simulink model "vd_controller"  (R2019b)
settings: configuration reference "E9_ECU_Configuration" (kept outside this file)
undefined symbols (not defined in the file or in its folder): BrakeMap_default_breakpoints, BrakeMap_default_data, disable_9D_front, disable_slipanglesensor, mask_select_input_pGL, Sq_PosBadGradient, Sq_PosIsFrozen, Sq_PosOutOfBounds
libraries: SignalProcessingSensorFusionLib x38, simulink x30, hdlsllib x3
(part 1 of 2)
settings Model: DataDictionary=dd_MainControl.sldd  EnableAccessToBaseWorkspace=off  ExplicitPartitioning=on  Creator=chwit  LastModifiedBy=laura
settings Model: ModifiedComment=|
  | schwa -- Fri Mar 02 10:09:33 2018 -- Version 1.53
  | Switched names of ControlAllocation, minimal Version active
settings Model: ModifiedHistory=|
  | schwa -- Fri Mar 02 10:09:33 2018 -- Version 1.53
  | Switched names of ControlAllocation, minimal Version active
  | 
  | schwa -- Fri Mar 02 10:09:33 2018 -- Version 1.53
  | Switched names of ControlAllocation, minimal Version active
  | 
  | schwa -- Fri Mar 02 01:32:20 2018 -- Version 1.52
  | cosmetic changes, adjusted ports
  | 
  | schwa -- Fri Mar 02 01:28:29 2018 -- Version 1.51
  | 
  | schwa -- Fri Mar 02 01:26:02 2018 -- Version 1.50
  | integrated new FF
  | 
  | 
  | chwit -- Fri Feb 23 19:55:57 2018 -- Version 1.49
  | 
  | chwit -- Fri Feb 23 07:06:27 2018 -- Version 1.48
  | Buildable but yet not flashable version of initial version of ControlSystem for E9 after function freeze v1
  | 
  | 
  | 
  | chwit -- Sun Feb 18 18:12:23 2018 -- Version 1.20
  | 
  | chwit -- Sun Feb 18 18:12:23 2018 -- Version 1.20
  | 
  | chwit -- Sun Feb 18 18:02:59 2018 -- Version 1.19
  | 
  | chwit -- Sun Feb 18 17:57:29 2018 -- Version 1.18
  | Saving
  | 
  | 
  | chwit -- Sun Feb 18 17:09:51 2018 -- Version 1.17
  | Saving
  | 
  | chwit -- Sun Feb 18 17:09:04 2018 -- Version 1.16
  | Just for saving purposes
  | 
  | chwit -- Sun Feb 18 14:38:44 2018 -- Version 1.15
  | YawMoment -> YawAcc corrected
  | 
  | 
  | chwit -- Sun Feb 18 12:57:57 2018 -- Version 1.14
  | Function freeze and new structure
  | 
  | 
  | chwit -- Sun Feb 18 12:51:11 2018 -- Version 1.13
  | Changes made due to function freeze and new structure
  | 
  | 
  | chwit -- Sun Feb 18 11:51:16 2018 -- Version 1.11
  | Implemented Manual Mode
  | 
  | chwit -- Sun Feb 18 11:51:16 2018 -- Version 1.11
  | Implemented Manual Mode
  | 
  | Marko -- Sat Feb 17 23:21:38 2018 -- Version 1.10
  | Changed Subsystem ConvertToInverterSingals: Deleted Everything except kt-Kennlinie, added limit on TorqueRequest
  | 
  | added OverUndersteerCorrection between FF and CA, connected CA with temporary (dummy) signals until right signals are provided
  | schwa -- Wed Feb 14 10:07:50 2018 -- Version 1.9
  | 
  | rearranged signals
  | schwa -- Wed Feb 14 09:51:50 2018 -- Version 1.8
  | 
  | chwit -- Sat Jan 20 18:54:27 2018 -- Version 1.7
  | 
  | chwit -- Sat Jan 20 17:46:44 2018 -- Version 1.6
  | 
  | chwit -- Sat Jan 20 17:42:35 2018 -- Version 1.5
  | Initial version
settings ConfigSetRef: SourceName=E9_ECU_Configuration

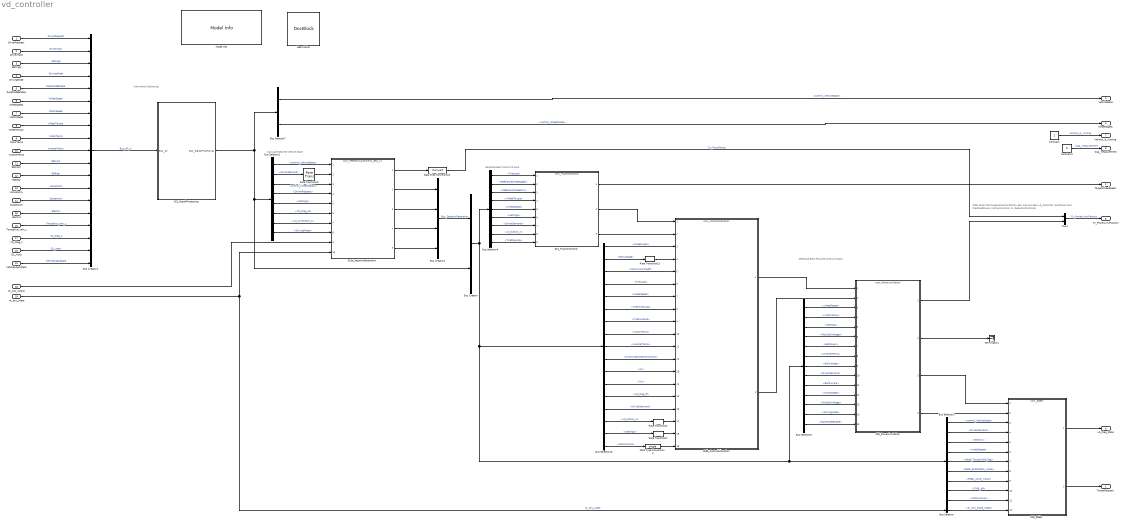
== system vd_controller ==
  note: ToDo: Einen Fahrzeugzustand einführen, den man aus dem
      |  vd_controller rausführen kann: PredictedPower, KalmanZustand, Fx, ReductionFaktoren
  note: Information Gathering
  note: Calculate Desired Vehicle State
  note: Generate Best Control Output
  note: Generate Best Possible Control Output
  DriverRequest : Inport  OutDataTypeStr=Bus: control_DriverRequest  SampleTime=0.01
  DriverInput : Inport  Port=2  OutDataTypeStr=Bus: control_DriverInput  SampleTime=0.1
  Settings : Inport  Port=3  OutDataTypeStr=Bus: control_Settings  SampleTime=0.1
  DrivingMode : Inport  Port=4  OutDataTypeStr=single  PortDimensions=1  SampleTime=0.1
  RaceModeEnable : Inport  Port=5  OutDataTypeStr=boolean  SampleTime=0.1
  WheelSpeed : Inport  Port=6  OutDataTypeStr=single  PortDimensions=4  SampleTime=0.001
  MotorSpeed : Inport  Port=7  OutDataTypeStr=single  PortDimensions=4  SampleTime=0.001
  WheelTorque : Inport  Port=8  OutDataTypeStr=single  PortDimensions=4  SampleTime=0.001
  MotorTemp : Inport  Port=9  OutDataTypeStr=single  PortDimensions=4  SampleTime=0.5
  InverterTemp : Inport  Port=10  OutDataTypeStr=single  PortDimensions=4  SampleTime=0.5
  9DFront : Inport  Port=11  OutDataTypeStr=Bus: control_9D  SampleTime=0.002
  9DRear : Inport  Port=12  OutDataTypeStr=Bus: control_9D  SampleTime=0.002
  v2oVelocity : Inport  Port=13  OutDataTypeStr=Bus: control_Velocity  SampleTime=0.004
  Suspension : Inport  Port=14  OutDataTypeStr=Bus: control_Suspension  SampleTime=0.01
  Electric : Inport  Port=15  OutDataTypeStr=Bus: control_Electric  SampleTime=0.005
  TorqueOut_raw_z : Inport  Port=16  OutDataTypeStr=single  PortDimensions=4  SampleTime=0.001
  VD_Diag_z : Inport  Port=17  OutDataTypeStr=uint32  SampleTime=0.001
  "dv_sdc_output " : Inport  Port=18  OutDataTypeStr=Bus: dv_sdc_output
  dv_ecu_state : Inport  Port=19  OutDataTypeStr=Bus: dv_ecu_state
  SiL_Input : Inport  Port=20  OutDataTypeStr=Bus: control_SiL_Input  SampleTime=0.002
  VehicleLogicState : Inport  Port=21  OutDataTypeStr=Bus: control_VehicleLogicState
  021_SignalProcessing : Subsystem
  "023a_SetpointGeneration  " : ModelReference  ModelNameDialog=com_FeedForwardControl_E10_v1.slx  SimulationMode=Normal  ModelReferenceVersion=1.405
  023b_ControlAllocation : ModelReference  ModelNameDialog=com_ControlAllocation.slx  SimulationMode=Normal  ModelReferenceVersion=1.474
  024_TractionControl : ModelReference  ModelNameDialog=com_TractionControl.slx  SimulationMode=Normal  ModelReferenceVersion=1.177
  025_PowerLimitation : ModelReference  ModelNameDialog=com_PowerLimitation.slx  SimulationMode=Normal  ModelReferenceVersion=1.281
  026_Safety : ModelReference  ModelNameDialog=com_Safety.slx  SimulationMode=Normal  ModelReferenceVersion=1.133
  Bus Creator : BusCreator  Inputs=2
  Bus Creator1 : BusCreator  Inputs=19
  Bus Creator2 : BusCreator  Inputs=4
  Bus Selector : BusSelector  OutputSignals=dv_ecu_state_state
  Bus Selector10 : BusSelector  OutputSignals=Bus_SignalProcessing.control_WheelStates.WheelAngle,Bus_SignalProcessing.electric.BatVoltage,Bus_SignalProcessing.control_WheelStates.MaxFrictionCoeff,Bus_SignalProcessing.control_WheelStates.TireLoad,Bus_SignalProcessing.wheelSpeed,Bus_SignalProcessing.control_WheelStates.TireForceLong,Bus_SignalProcessing.control_WheelStates.TireForceLat,Bus_SignalProcessing.motorTemp,Bus_SignalProcessing.inverterTemp,Bus_SetpointGeneration.OverUndersteerCorrection,Bus_SetpointGeneration.Fx,Bus_SetpointGeneration.Mz,Bus_SetpointGeneration.VD_Diag_ff,Bus_SignalProcessing.DriverDemand,Bus_SignalProcessing.HMI_DriverNotice.vd_button_2,Bus_SignalProcessing.settings,Bus_SignalProcessing.VehicleLogicState.MotorActive
  Bus Selector2 : BusSelector  OutputSignals=control_VehicleState,DriverDemand,control_WheelStates,DriverRequest,settings,VD_Diag_sf,HMI_DriverNotice.vd_turnbutton_2,HMI_DriverNotice.DrivingMode
  Bus Selector3 : BusSelector  OutputSignals=Bus_SignalProcessing.control_VehicleState,Bus_SignalProcessing.DriverDemand,Bus_SignalProcessing.electric,Bus_SignalProcessing.wheelSpeed,Bus_SignalProcessing.DriverRequest.Pedal_TorqueValid_flag,Bus_SignalProcessing.DriverRequest.Pedal_BrakeMech_Value,Bus_SignalProcessing.DriverRequest.Pedal_Accel_Value,Bus_SignalProcessing.settings.TWB_off,Bus_SignalProcessing.VehicleLogicState.MotorActive
  Bus Selector4 : BusSelector  OutputSignals=Bus_SignalProcessing.control_WheelStates.TireLoad,Bus_SignalProcessing.control_WheelStates.ReferenceWheelSpeed,Bus_SignalProcessing.control_WheelStates.ReferenceWheelAcc,Bus_SignalProcessing.WheelTorque,Bus_SignalProcessing.wheelSpeed,Bus_SignalProcessing.settings,Bus_SignalProcessing.DriverDemand,Bus_SignalProcessing.HMI_DriverNotice.vd_button_2,Bus_SignalProcessing.control_WheelStates.TireSlipLong
  Bus Selector5 : BusSelector  OutputSignals=Bus_SignalProcessing.wheelSpeed,Bus_SignalProcessing.motorTemp,Bus_SignalProcessing.settings,Bus_SignalProcessing.electric.MaxCellVoltage,Bus_SignalProcessing.electric.BatPower,Bus_SignalProcessing.inverterTemp,Bus_SignalProcessing.electric.BatVoltage,Bus_SignalProcessing.DriverDemand,Bus_SignalProcessing.electric.BatCurrent,Bus_SignalProcessing.motorSpeed,Bus_SignalProcessing.electric.MinCellVoltage,Bus_SignalProcessing.HMI_DriverNotice.DrivingMode,Bus_SignalProcessing.RaceModeEnable
  Bus Selector7 : BusSelector  OutputSignals=control_VehicleState,control_WheelStates
  Constant : Constant
  Constant1 : Constant  Value=0  OutDataTypeStr=boolean
  Data Type Conversion2 : DataTypeConversion
  Data Type Conversion4 : DataTypeConversion  OutDataTypeStr=single
  Description : simulink/Model-Wide Utilities/DocBlock  DocumentType=Text
      content=|
      | Beschreibung:
      |
      | Schlupfsollwert wird über Settings-Protokoll vorgegeben. Wird entsprechend mit Vorzeichen Torque-Request verrechnet.
      | Desgin-Parameter sind Lyap_kp (nützlich, linearer Faktor) und Lyap_p (nicht so nützlich, Potenz -> sollte ungerade sein (nicht ganz sicher)).
      |
      | I-Anteil mit Anti-WindUp zur Verbesserung Regler und Stellgrößenbeschränkung vorzubeugen.
      |
      | Tiefpassfilter (PT1) zur Verminderung von Schwingungen.
      |
      | Lambda_mux ist der Einstellparameter für den Reibwert, mit dem das SetUp stark verändert werden kann.
      |
      | Multiport-Switches zur Auswahl diverser Ansätze für die Traktionskontrolle bzw. zur Abschaltung.
      |
      | Adaptive_RG Schlupfgeschw.: adaptiver Regler mit Reibwerschätzer, schätzt Reibwert und regelt entsprechend Schlupf
      |     -> hat nicht wirklich funktioniert, Schätzen war wohl schon scheiße, Konzept fragwürdig
      |
      | LQRI: Linearisierter Lyap. Regler mit diversen Betriebspunkten (Gain-Scheduling), ähnliche Gleichungen wie Lyap
      |     -> durch Linearisierung etwas schlechter als Lyap
  Model Info : simulink/Model-Wide Utilities/Model Info  Frame=on  DisplayStringWithTags=|  HorizontalTextAlignment=Center  LeftAlignmentValue=0.5
      | Model Name: %<ModelName>
      | Responsible: Christian Witte
      | 
      | Last modified by: %<LastModifiedBy>
      | Last modified: %<LastModificationDate>
      | Current Version: %<ModelVersion>
  Mux2 : Mux  Inputs=2
  Rate Transition{1..3,13} (4 alike) : RateTransition  Deterministic=off  OutPortSampleTime=0.001
  Terminator1 : Terminator
  TorqueRequest : Outport  OutDataTypeStr=single  PortDimensions=4  VectorParamsAs1DForOutWhenUnconnected=off
  TargetWheelSpeed : Outport  Port=2  OutDataTypeStr=single  PortDimensions=4  VectorParamsAs1DForOutWhenUnconnected=off
  VehicleState : Outport  Port=3  OutDataTypeStr=Bus: control_VehicleState  VectorParamsAs1DForOutWhenUnconnected=off
  WheelStates : Outport  Port=4  OutDataTypeStr=Bus: control_WheelStates  VectorParamsAs1DForOutWhenUnconnected=off
  Fx_PowerLimitFactors : Outport  Port=5  OutDataTypeStr=single  PortDimensions=3  VectorParamsAs1DForOutWhenUnconnected=off
  vd_Diag_State : Outport  Port=6  OutDataTypeStr=uint32  PortDimensions=1  VectorParamsAs1DForOutWhenUnconnected=off
  kalman_is_running : Outport  Port=7  VectorParamsAs1DForOutWhenUnconnected=off
  bias_measurement : Outport  Port=8  VectorParamsAs1DForOutWhenUnconnected=off
  wires:
  025_PowerLimitation/2 -> Terminator1/1
  Bus Creator1/1 -> 021_SignalProcessing/1(Bus_all)  "Bus_all_in"
  Bus Creator2/1 -> Bus Creator/1  "Bus_SetpointGeneration"
  021_SignalProcessing/1(Bus_SignalProcessing) -> Bus Selector7/1, Bus Creator/2, Bus Selector2/1
  Bus Selector5/1 -> 025_PowerLimitation/3  "<wheelSpeed>"
  Bus Selector5/2 -> 025_PowerLimitation/4  "<motorTemp>"
  Bus Selector5/3 -> 025_PowerLimitation/5  "<settings>"
  Bus Selector5/4 -> 025_PowerLimitation/6  "<MaxCellVoltage>"
  Bus Selector5/5 -> 025_PowerLimitation/7  "<BatPower>"
  Bus Selector5/6 -> 025_PowerLimitation/8  "<inverterTemp>"
  Bus Selector5/7 -> 025_PowerLimitation/9  "<BatVoltage>"
  Bus Selector5/8 -> 025_PowerLimitation/10  "<DriverDemand>"
  Bus Selector3/1 -> 026_Safety/3  "<control_VehicleState>"
  Bus Selector3/2 -> 026_Safety/4  "<DriverDemand>"
  Bus Selector3/3 -> 026_Safety/5  "<electric>"
  Bus Selector3/4 -> 026_Safety/6  "<wheelSpeed>"
  Bus Selector3/5 -> 026_Safety/7  "<Pedal_TorqueValid_flag>"
  025_PowerLimitation/4 -> 026_Safety/2
  Bus Selector10/1 -> 023b_ControlAllocation/3  "<WheelAngle>"
  Bus Selector10/2 -> Rate Transition13/1  "<BatVoltage>"
  Bus Selector10/3 -> 023b_ControlAllocation/5  "<MaxFrictionCoeff>"
  Bus Selector10/4 -> 023b_ControlAllocation/6  "<TireLoad>"
  Bus Selector10/10 -> 023b_ControlAllocation/12  "<OverUndersteerCorrection>"
  Bus Selector10/11 -> 023b_ControlAllocation/13  "<Fx>"
  026_Safety/2 -> TorqueRequest/1
  026_Safety/1 -> vd_Diag_State/1
  Bus Selector4/7 -> 024_TractionControl/7  "<DriverDemand>"
  Bus Selector4/6 -> 024_TractionControl/6  "<settings>"
  Bus Selector4/5 -> 024_TractionControl/5  "<wheelSpeed>"
  Bus Selector4/4 -> 024_TractionControl/4  "<WheelTorque>"
  Bus Selector4/3 -> 024_TractionControl/3  "<ReferenceWheelAcc>"
  Bus Selector10/13 -> 023b_ControlAllocation/15  "<VD_Diag_ff>"
  Bus Selector10/6 -> 023b_ControlAllocation/8  "<TireForceLong>"
  Bus Selector10/7 -> 023b_ControlAllocation/9  "<TireForceLat>"
  9DFront/1 -> Bus Creator1/11  "9DFront"
  9DRear/1 -> Bus Creator1/12  "9DRear"
  v2oVelocity/1 -> Bus Creator1/13  "v2oVelocity"
  Suspension/1 -> Bus Creator1/14  "Suspension"
  DriverRequest/1 -> Bus Creator1/1  "DriverRequest"
  TorqueOut_raw_z/1 -> Bus Creator1/16  "TorqueOut_raw_z"
  Electric/1 -> Bus Creator1/15  "Electric"
  VD_Diag_z/1 -> Bus Creator1/17  "VD_Diag_z"
  WheelSpeed/1 -> Bus Creator1/6  "WheelSpeed"
  MotorSpeed/1 -> Bus Creator1/7  "MotorSpeed"
  WheelTorque/1 -> Bus Creator1/8  "WheelTorque"
  MotorTemp/1 -> Bus Creator1/9  "MotorTemp"
  InverterTemp/1 -> Bus Creator1/10  "InverterTemp"
  Settings/1 -> Bus Creator1/3  "Settings"
  DriverInput/1 -> Bus Creator1/2  "DriverInput"
  Bus Selector2/1 -> "023a_SetpointGeneration  "/1  "<control_VehicleState>"
  Bus Selector2/2 -> Rate Transition3/1  "<DriverDemand>"
  Bus Selector2/3 -> "023a_SetpointGeneration  "/3  "<control_WheelStates>"
  Bus Selector2/4 -> "023a_SetpointGeneration  "/4  "<DriverRequest>"
  Bus Selector2/5 -> "023a_SetpointGeneration  "/5  "<settings>"
  Bus Selector2/6 -> "023a_SetpointGeneration  "/6  "<VD_Diag_sf>"
  Bus Selector5/9 -> 025_PowerLimitation/11  "<BatCurrent>"
  Bus Selector3/6 -> 026_Safety/8  "<Pedal_BrakeMech_Value>"
  Bus Selector3/7 -> 026_Safety/9  "<Pedal_Accel_Value>"
  SiL_Input/1 -> Bus Creator1/18  "SiL_Input"
  Bus Selector10/14 -> 023b_ControlAllocation/16  "<DriverDemand>"
  Bus Selector5/10 -> 025_PowerLimitation/12  "<motorSpeed>"
  Rate Transition3/1 -> "023a_SetpointGeneration  "/2
  DrivingMode/1 -> Bus Creator1/4  "DrivingMode"
  Bus Selector5/12 -> 025_PowerLimitation/14  "<DrivingMode>"
  Bus Selector5/11 -> 025_PowerLimitation/13  "<MinCellVoltage>"
  Bus Selector4/8 -> 024_TractionControl/8  "<vd_button_2>"
  Bus Selector2/7 -> "023a_SetpointGeneration  "/7  "<vd_turnbutton_2>"
  Bus Selector10/15 -> Rate Transition2/1  "<vd_button_2>"
  Bus Selector10/16 -> Rate Transition1/1  "<settings>"
  Bus Selector2/8 -> "023a_SetpointGeneration  "/8  "<DrivingMode>"
  RaceModeEnable/1 -> Bus Creator1/5  "RaceModeEnable"
  Bus Selector3/8 -> 026_Safety/10  "<TWB_off>"
  Bus Selector10/12 -> 023b_ControlAllocation/14  "<Mz>"
  025_PowerLimitation/1 -> Mux2/2
  Mux2/1 -> Fx_PowerLimitFactors/1  "Fx_PowerLimitFactors"
  "023a_SetpointGeneration  "/1 -> Data Type Conversion2/1
  Bus Selector4/2 -> 024_TractionControl/2  "<ReferenceWheelSpeed>"
  Bus Selector4/1 -> 024_TractionControl/1  "<TireLoad>"
  023b_ControlAllocation/2 -> 025_PowerLimitation/2
  024_TractionControl/2 -> 023b_ControlAllocation/1
  024_TractionControl/3 -> 023b_ControlAllocation/2
  Rate Transition13/1 -> 023b_ControlAllocation/4
  Bus Selector10/5 -> 023b_ControlAllocation/7  "<wheelSpeed>"
  Bus Selector10/8 -> 023b_ControlAllocation/10  "<motorTemp>"
  Bus Selector10/9 -> 023b_ControlAllocation/11  "<inverterTemp>"
  023b_ControlAllocation/1 -> 025_PowerLimitation/1
  Bus Selector4/9 -> 024_TractionControl/9  "<TireSlipLong>"
  Data Type Conversion4/1 -> 023b_ControlAllocation/19
  VehicleLogicState/1 -> Bus Creator1/19  "VehicleLogicState"
  Bus Selector10/17 -> Data Type Conversion4/1  "<MotorActive>"
  Bus Selector3/9 -> 026_Safety/11  "<MotorActive>"
  Bus Selector7/1 -> VehicleState/1  "<control_VehicleState>"
  Bus Selector7/2 -> WheelStates/1  "<control_WheelStates>"
  024_TractionControl/1 -> TargetWheelSpeed/1
  Bus Creator/1 -> Bus Selector4/1, Bus Selector10/1, Bus Selector3/1, Bus Selector5/1
  025_PowerLimitation/3 -> 026_Safety/1
  Bus Selector5/13 -> 025_PowerLimitation/15  "<RaceModeEnable>"
  Rate Transition1/1 -> 023b_ControlAllocation/18
  Rate Transition2/1 -> 023b_ControlAllocation/17
  Constant/1 -> kalman_is_running/1  "kalman_is_running"
  Constant1/1 -> bias_measurement/1  "bias_measurement"
  dv_ecu_state/1 -> Bus Selector/1, "023a_SetpointGeneration  "/10  "dv_ecu_state"
  "dv_sdc_output "/1 -> "023a_SetpointGeneration  "/9
  "023a_SetpointGeneration  "/2 -> Bus Creator2/1
  "023a_SetpointGeneration  "/3 -> Bus Creator2/2
  "023a_SetpointGeneration  "/4 -> Bus Creator2/3
  "023a_SetpointGeneration  "/5 -> Bus Creator2/4
  Data Type Conversion2/1 -> Mux2/1  "Fx_ForceFactor"
  Bus Selector/1 -> 026_Safety/12  "<dv_ecu_state_state>"

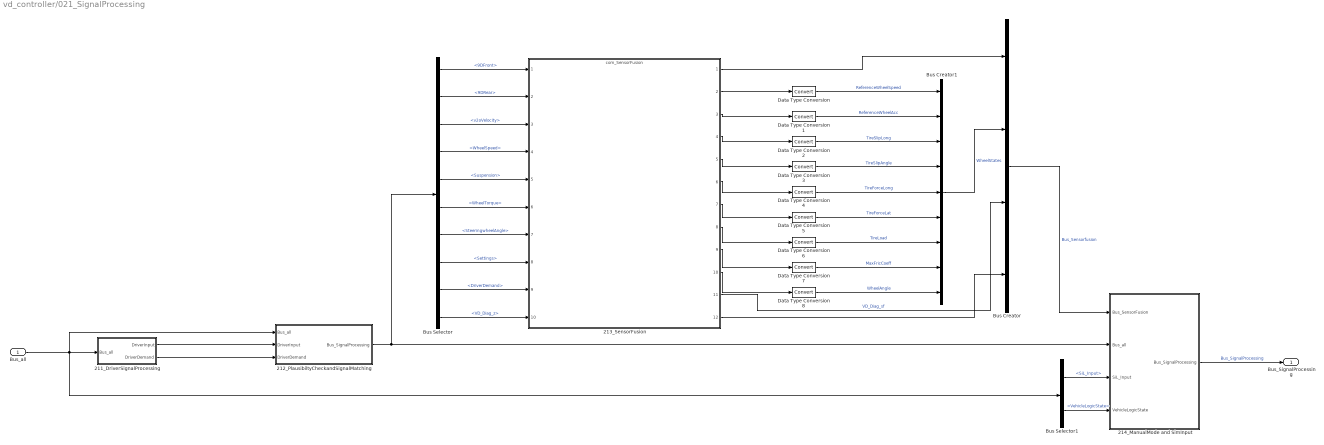
== system vd_controller/021_SignalProcessing ==
  Bus_all : Inport
  211_DriverSignalProcessing : Subsystem
  212_PlausibiltyCheckandSignalMatching : Subsystem
  213_SensorFusion : ModelReference  ModelNameDialog=com_SensorFusion.slx  SimulationMode=Normal  ModelReferenceVersion=1.609
  214_ManualMode and SimInput : Subsystem
  Bus Creator : BusCreator  Inputs=4
  Bus Creator1 : BusCreator  Inputs=9
  Bus Selector : BusSelector  OutputSignals=9DFront,9DRear,v2oVelocity,WheelSpeed,Suspension,WheelTorque,DriverRequest.SteeringwheelAngle,Settings,DriverDemand,VD_Diag_z
  Bus Selector1 : BusSelector  OutputSignals=SiL_Input,VehicleLogicState
  Data Type Conversion{,1..8} (9 alike) : DataTypeConversion
  Bus_SignalProcessing : Outport  VectorParamsAs1DForOutWhenUnconnected=off
  wires:
  213_SensorFusion/1 -> Bus Creator/1
  Bus Creator/1 -> 214_ManualMode and SimInput/1(Bus_SensorFusion)  "Bus_Sensorfusion"
  Bus Selector/5 -> 213_SensorFusion/5  "<Suspension>"
  Bus Selector/2 -> 213_SensorFusion/2  "<9DRear>"
  Bus Selector/3 -> 213_SensorFusion/3  "<v2oVelocity>"
  Bus Selector/1 -> 213_SensorFusion/1  "<9DFront>"
  Bus Selector/4 -> 213_SensorFusion/4  "<WheelSpeed>"
  Bus Selector/6 -> 213_SensorFusion/6  "<WheelTorque>"
  212_PlausibiltyCheckandSignalMatching/1(Bus_SignalProcessing) -> 214_ManualMode and SimInput/2(Bus_all), Bus Selector/1
  Bus Selector1/1 -> 214_ManualMode and SimInput/3(SiL_Input)  "<SiL_Input>"
  213_SensorFusion/6 -> Data Type Conversion4/1
  213_SensorFusion/5 -> Data Type Conversion3/1
  213_SensorFusion/3 -> Data Type Conversion1/1
  213_SensorFusion/4 -> Data Type Conversion2/1
  213_SensorFusion/7 -> Data Type Conversion5/1
  213_SensorFusion/8 -> Data Type Conversion6/1
  Bus Creator1/1 -> Bus Creator/2  "WheelStates"
  Data Type Conversion3/1 -> Bus Creator1/4  "TireSlipAngle"
  Data Type Conversion2/1 -> Bus Creator1/3  "TireSlipLong"
  Data Type Conversion/1 -> Bus Creator1/1  "ReferenceWheelSpeed"
  Data Type Conversion6/1 -> Bus Creator1/7  "TireLoad"
  Data Type Conversion4/1 -> Bus Creator1/5  "TireForceLong"
  Data Type Conversion7/1 -> Bus Creator1/8  "MaxFricCoeff"
  Data Type Conversion5/1 -> Bus Creator1/6  "TireForceLat"
  Data Type Conversion1/1 -> Bus Creator1/2  "ReferenceWheelAcc"
  213_SensorFusion/2 -> Data Type Conversion/1
  213_SensorFusion/9 -> Data Type Conversion7/1
  Bus Selector/8 -> 213_SensorFusion/8  "<Settings>"
  Bus Selector/7 -> 213_SensorFusion/7  "<SteeringwheelAngle>"
  213_SensorFusion/10 -> Data Type Conversion8/1
  Data Type Conversion8/1 -> Bus Creator1/9  "WheelAngle"
  Bus Selector1/2 -> 214_ManualMode and SimInput/4(VehicleLogicState)  "<VehicleLogicState>"
  214_ManualMode and SimInput/1(Bus_SignalProcessing) -> Bus_SignalProcessing/1  "Bus_SignalProcessing"
  Bus Selector/9 -> 213_SensorFusion/9  "<DriverDemand>"
  213_SensorFusion/11 -> Bus Creator/3  "VD_Diag_sf"
  211_DriverSignalProcessing/1(DriverInput) -> 212_PlausibiltyCheckandSignalMatching/2(DriverInput)
  211_DriverSignalProcessing/2(DriverDemand) -> 212_PlausibiltyCheckandSignalMatching/3(DriverDemand)
  Bus Selector/10 -> 213_SensorFusion/10  "<VD_Diag_z>"
  Bus_all/1 -> 212_PlausibiltyCheckandSignalMatching/1(Bus_all), 211_DriverSignalProcessing/1(Bus_all), Bus Selector1/1
  213_SensorFusion/12 -> Bus Creator/4

== system vd_controller/021_SignalProcessing/211_DriverSignalProcessing ==
  Bus_all : Inport
  Bus Selector : BusSelector  OutputSignals=DriverInput,DrivingMode,DriverRequest,DriverInput.driver
  Bus Selector2 : BusSelector  OutputSignals=Pedal_BrakeRecu_Value,Pedal_BrakeMech_Value,Pedal_Accel_Value
  DriverDemand_Generation_LaunchControl : Subsystem
  DriverInput_Generation : Subsystem
  DriverInput : Outport  VectorParamsAs1DForOutWhenUnconnected=off
  DriverDemand : Outport  Port=2  VectorParamsAs1DForOutWhenUnconnected=off
  wires:
  Bus Selector/1 -> DriverInput_Generation/1(DriverInput_in)  "<DriverInput>"
  DriverInput_Generation/1(DriverInput) -> DriverInput/1
  Bus_all/1 -> Bus Selector/1
  Bus Selector2/3 -> DriverDemand_Generation_LaunchControl/4(PedalAccelValue)  "<Pedal_Accel_Value>"
  Bus Selector2/2 -> DriverDemand_Generation_LaunchControl/3(Pedal_BrakeMechValue)  "<Pedal_BrakeMech_Value>"
  Bus Selector/4 -> DriverDemand_Generation_LaunchControl/5(Driver)  "<driver>"
  DriverDemand_Generation_LaunchControl/1(DriverDemand) -> DriverDemand/1
  Bus Selector/2 -> DriverDemand_Generation_LaunchControl/1(DrivingMode), DriverInput_Generation/2(DrivingMode)  "<DrivingMode>"
  Bus Selector2/1 -> DriverDemand_Generation_LaunchControl/2(PedalBrakeRecuValue)  "<Pedal_BrakeRecu_Value>"
  Bus Selector/3 -> Bus Selector2/1  "<DriverRequest>"

== system vd_controller/021_SignalProcessing/212_PlausibiltyCheckandSignalMatching ==
  Bus_all : Inport
  DriverInput : Inport  Port=2
  DriverDemand : Inport  Port=3
  9DFront_Plausibility : Subsystem
  9DRear_Plausibility : Subsystem
  Bus Creator1 : BusCreator  Inputs=21
  Bus Selector1 : BusSelector  OutputSignals=9DFront,9DRear,Settings,v2oVelocity,WheelSpeed,Suspension,Electric,WheelTorque,MotorTemp,InverterTemp,MotorSpeed,DriverRequest,VD_Diag_z,TorqueOut_raw_z,RaceModeEnable
  DriverRequest_Plausibility : Subsystem
  Electric_Plausibility : Subsystem
  InverterTemp_Plausibility : Subsystem
  MotorSpeed_Plausibility : Subsystem
  MotorTemp_Plausibility : Subsystem
  Suspension_Plausibility : Subsystem
  WheelSpeed_Plausibility : Subsystem
  v2oVelocity_Plausibility : Subsystem
  Bus_SignalProcessing : Outport  VectorParamsAs1DForOutWhenUnconnected=off
  wires:
  Bus Selector1/5 -> WheelSpeed_Plausibility/1(In)  "<WheelSpeed>"
  Bus Selector1/4 -> v2oVelocity_Plausibility/1(In)  "<v2oVelocity>"
  Bus_all/1 -> Bus Selector1/1
  Bus Selector1/8 -> Bus Creator1/9  "<WheelTorque>"
  Bus Creator1/1 -> Bus_SignalProcessing/1  "Bus_all"
  Bus Selector1/2 -> 9DRear_Plausibility/1(In)  "<9DRear>"
  Bus Selector1/6 -> Suspension_Plausibility/1(In)  "<Suspension>"
  Bus Selector1/7 -> Electric_Plausibility/1(In)  "<Electric>"
  Bus Selector1/3 -> Bus Creator1/3  "<Settings>"
  Bus Selector1/9 -> MotorTemp_Plausibility/1(In)  "<MotorTemp>"
  Bus Selector1/11 -> MotorSpeed_Plausibility/1(In)  "<MotorSpeed>"
  Bus Selector1/12 -> DriverRequest_Plausibility/1(In)  "<DriverRequest>"
  Bus Selector1/1 -> 9DFront_Plausibility/1(In)  "<9DFront>"
  9DFront_Plausibility/1(9DFrontPlausible) -> Bus Creator1/1  "9DFront"
  9DRear_Plausibility/1(9DRearPlausible) -> Bus Creator1/2  "9DRear"
  v2oVelocity_Plausibility/1(v2oVelocityPlausible) -> Bus Creator1/4  "v2oVelocity"
  WheelSpeed_Plausibility/1(WheelSpeedPlausible) -> Bus Creator1/5  "WheelSpeed"
  Suspension_Plausibility/1(SuspensionPlausible) -> Bus Creator1/7  "Suspension"
  MotorSpeed_Plausibility/1(MotorSpeed) -> Bus Creator1/14  "MotorSpeed"
  Bus Selector1/10 -> InverterTemp_Plausibility/1(In)  "<InverterTemp>"
  DriverRequest_Plausibility/1(DriverRequest) -> Bus Creator1/16  "DriverRequest"
  Electric_Plausibility/1(ElectricPlausible) -> Bus Creator1/8  "Electric"
  WheelSpeed_Plausibility/2(WheelSpeed_Sq) -> Bus Creator1/6  "WheelSpeed_Sq"
  MotorSpeed_Plausibility/2(MotorSpeed_Sq) -> Bus Creator1/15  "MotorSpeed_Sq"
  MotorTemp_Plausibility/1(MotorTempPlausible) -> Bus Creator1/10  "MotorTemp"
  MotorTemp_Plausibility/2(MotorTemp_Sq) -> Bus Creator1/11  "MotorTemp_Sq"
  InverterTemp_Plausibility/1(InverterTempPlausible) -> Bus Creator1/12  "InverterTemp"
  InverterTemp_Plausibility/2(InverterTemp_Sq) -> Bus Creator1/13  "InverterTemp_Sq"
  Bus Selector1/15 -> Bus Creator1/19  "<RaceModeEnable>"
  Bus Selector1/13 -> Bus Creator1/17  "<VD_Diag_z>"
  Bus Selector1/14 -> Bus Creator1/18  "<TorqueOut_raw_z>"
  DriverInput/1 -> Bus Creator1/20
  DriverDemand/1 -> Bus Creator1/21

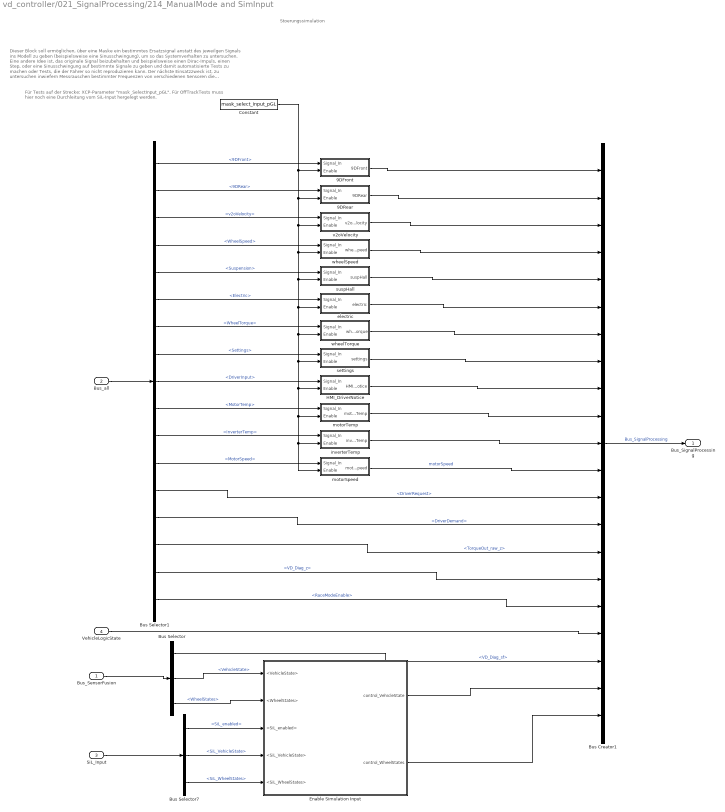
== system vd_controller/021_SignalProcessing/214_ManualMode and SimInput ==
  note: Stoerungssimulation
  note: Für Tests auf der Strecke: XCP-Parameter "mask_SelectInput_pGL".
      | Für OffTrackTests muss hier noch eine Durchleitung vom SiL-Input hergelegt werden.
  note: Dieser Block soll ermöglichen, über eine Maske ein bestimmtes Ersatzsignal anstatt des jeweilgen Signals ins Modell zu geben (beispielsweise eine Sinusschwingung), um so das Systemverhalten zu untersuchen.
      | Eine andere Idee ist, das originale Signal beizubehalten und beispielsweise einen Dirac-Impuls, einen Step, oder eine Sinusschwingung auf bestimmte Signale zu geben und damit automatisierte Tests zu machen oder Tests, die der Fahrer so nicht reproduzieren kann.
      | Der nächste Einsatzzweck ist, zu untersuchen inwiefern Messrauschen bestimmter Frequenzen von verschiedenen Sensoren die Momentenverteilung und den Momentenverlauf beeinflussen.
      | Hier können auch SiSO-Übertragungsfunktionen von den ausgewählten Sensoriksignalen auf die einzelnen Raddrehmomente gebildet werden. Idealerweise fallen diese dann zu hohen Frequenzen hin schnell ab, um keine Fahrzeugschwingungen zu induzieren.
  Bus_SensorFusion : Inport
  Bus_all : Inport  Port=2
  SiL_Input : Inport  Port=3
  VehicleLogicState : Inport  Port=4
  9DFront : Subsystem
  9DRear : Subsystem
  Bus Creator1 : BusCreator  Inputs=21
  Bus Selector : BusSelector  OutputSignals=VD_Diag_sf,VehicleState,WheelStates
  Bus Selector1 : BusSelector  OutputSignals=9DFront,9DRear,v2oVelocity,WheelSpeed,Suspension,Electric,WheelTorque,Settings,DriverInput,MotorTemp,InverterTemp,MotorSpeed,DriverRequest,DriverDemand,TorqueOut_raw_z,VD_Diag_z,RaceModeEnable
  Bus Selector7 : BusSelector  OutputSignals=SiL_enabled,SiL_VehicleState,SiL_WheelStates
  Constant : Constant  Value=mask_select_input_pGL
  Enable Simulation Input : Subsystem
  HMI_DriverNotice : Subsystem
  electric : Subsystem
  inverterTemp : Subsystem
  motorSpeed : Subsystem
  motorTemp : Subsystem
  settings : Subsystem
  suspHall : Subsystem
  v2oVelocity : Subsystem
  wheelSpeed : Subsystem
  wheelTorque : Subsystem
  Bus_SignalProcessing : Outport  VectorParamsAs1DForOutWhenUnconnected=off
  wires:
  Bus_SensorFusion/1 -> Bus Selector/1
  settings/1(settings) -> Bus Creator1/8
  wheelTorque/1(wheelTorque) -> Bus Creator1/7
  electric/1(electric) -> Bus Creator1/6
  suspHall/1(suspHall) -> Bus Creator1/5
  wheelSpeed/1(wheelSpeed) -> Bus Creator1/4
  v2oVelocity/1(v2oVelocity) -> Bus Creator1/3
  9DRear/1(9DRear) -> Bus Creator1/2
  9DFront/1(9DFront) -> Bus Creator1/1
  Constant/1 -> v2oVelocity/2(Enable), suspHall/2(Enable), motorSpeed/2(Enable), inverterTemp/2(Enable), motorTemp/2(Enable), HMI_DriverNotice/2(Enable), settings/2(Enable), wheelTorque/2(Enable), electric/2(Enable), wheelSpeed/2(Enable), 9DRear/2(Enable), 9DFront/2(Enable)
  Bus Selector1/13 -> Bus Creator1/13  "<DriverRequest>"
  Bus Selector1/10 -> motorTemp/1(Signal_In)  "<MotorTemp>"
  Bus Selector1/11 -> inverterTemp/1(Signal_In)  "<InverterTemp>"
  Bus Selector1/12 -> motorSpeed/1(Signal_In)  "<MotorSpeed>"
  Bus Selector1/4 -> wheelSpeed/1(Signal_In)  "<WheelSpeed>"
  Bus Selector1/3 -> v2oVelocity/1(Signal_In)  "<v2oVelocity>"
  Bus_all/1 -> Bus Selector1/1
  Bus Selector1/7 -> wheelTorque/1(Signal_In)  "<WheelTorque>"
  Bus Selector1/9 -> HMI_DriverNotice/1(Signal_In)  "<DriverInput>"
  Bus Selector1/1 -> 9DFront/1(Signal_In)  "<9DFront>"
  Bus Creator1/1 -> Bus_SignalProcessing/1  "Bus_SignalProcessing"
  Bus Selector1/8 -> settings/1(Signal_In)  "<Settings>"
  Bus Selector1/2 -> 9DRear/1(Signal_In)  "<9DRear>"
  Bus Selector1/5 -> suspHall/1(Signal_In)  "<Suspension>"
  Bus Selector1/6 -> electric/1(Signal_In)  "<Electric>"
  HMI_DriverNotice/1(HMI_DriverNotice) -> Bus Creator1/9
  motorTemp/1(motorTemp) -> Bus Creator1/10
  inverterTemp/1(inverterTemp) -> Bus Creator1/11
  Bus Selector1/14 -> Bus Creator1/14  "<DriverDemand>"
  Bus Selector1/15 -> Bus Creator1/15  "<TorqueOut_raw_z>"
  Bus Selector1/16 -> Bus Creator1/16  "<VD_Diag_z>"
  SiL_Input/1 -> Bus Selector7/1
  Bus Selector1/17 -> Bus Creator1/17  "<RaceModeEnable>"
  VehicleLogicState/1 -> Bus Creator1/18
  Bus Selector/1 -> Bus Creator1/19  "<VD_Diag_sf>"
  Bus Selector/2 -> Enable Simulation Input/1(<VehicleState>)  "<VehicleState>"
  Bus Selector/3 -> Enable Simulation Input/2(<WheelStates>)  "<WheelStates>"
  Bus Selector7/2 -> Enable Simulation Input/4(<SiL_VehicleState>)  "<SiL_VehicleState>"
  Enable Simulation Input/1(control_VehicleState) -> Bus Creator1/20
  Enable Simulation Input/2(control_WheelStates) -> Bus Creator1/21
  Bus Selector7/3 -> Enable Simulation Input/5(<SiL_WheelStates>)  "<SiL_WheelStates>"
  Bus Selector7/1 -> Enable Simulation Input/3(<SiL_enabled>)  "<SiL_enabled>"
  motorSpeed/1(motorSpeed) -> Bus Creator1/12  "motorSpeed"

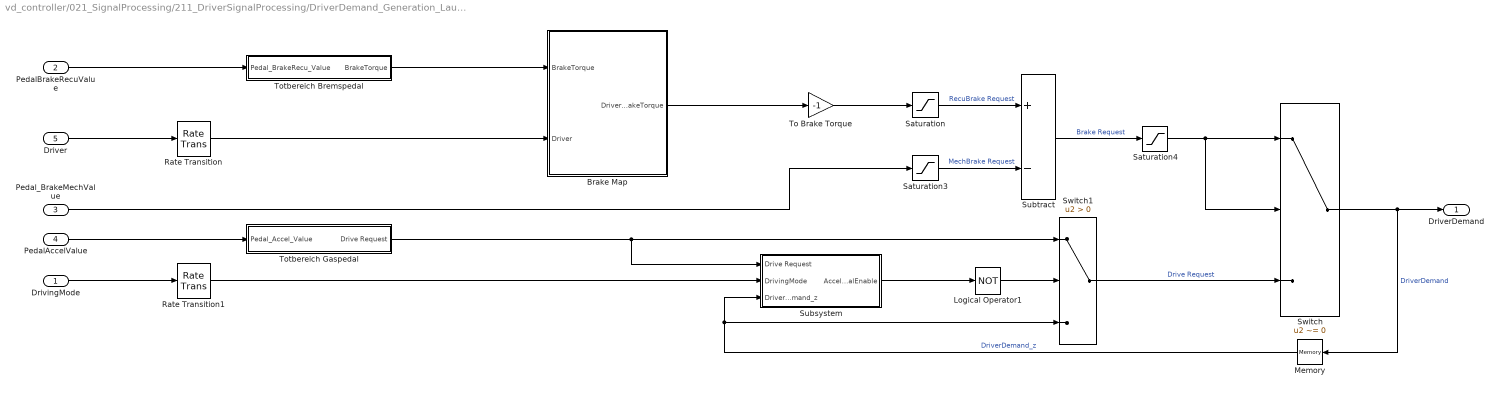
== system vd_controller/021_SignalProcessing/211_DriverSignalProcessing/DriverDemand_Generation_LaunchControl ==
  DrivingMode : Inport
  PedalBrakeRecuValue : Inport  Port=2
  Pedal_BrakeMechValue : Inport  Port=3
  PedalAccelValue : Inport  Port=4
  Driver : Inport  Port=5
  Brake Map : Subsystem
  Logical Operator1 : Logic  Operator=NOT  AllPortsSameDT=off  OutDataTypeStr=boolean
  Memory : Memory  InheritSampleTime=on
  Rate Transition : RateTransition  OutPortSampleTime=0.01
  Rate Transition1 : RateTransition  OutPortSampleTime=0.01
  Saturation : Saturate  UpperLimit=0  LowerLimit=-1
  Saturation3 : Saturate  UpperLimit=1  LowerLimit=0
  Saturation4 : Saturate  UpperLimit=0  LowerLimit=-2
  Subsystem : Subsystem
  Subtract : Sum  Inputs=+-
  Switch : Switch  Criteria=u2 ~= 0
  Switch1 : Switch  Criteria=u2 > Threshold
  To Brake Torque : Gain  Gain=-1
  Totbereich Bremspedal : Subsystem
  Totbereich Gaspedal : Subsystem
  DriverDemand : Outport  VectorParamsAs1DForOutWhenUnconnected=off
  wires:
  Switch/1 -> DriverDemand/1, Memory/1  "DriverDemand"
  Switch1/1 -> Switch/3  "Drive Request"
  Subtract/1 -> Saturation4/1  "Brake Request"
  To Brake Torque/1 -> Saturation/1
  Brake Map/1(DriverBrakeTorque) -> To Brake Torque/1
  Driver/1 -> Rate Transition/1
  Saturation/1 -> Subtract/1  "RecuBrake Request"
  Pedal_BrakeMechValue/1 -> Saturation3/1
  Saturation3/1 -> Subtract/2  "MechBrake Request"
  Saturation4/1 -> Switch/2, Switch/1
  Memory/1 -> Subsystem/3(DriverDemand_z), Switch1/3  "DriverDemand_z"
  DrivingMode/1 -> Rate Transition1/1
  Subsystem/1(AccelPedalEnable) -> Logical Operator1/1
  Totbereich Gaspedal/1(Drive Request) -> Subsystem/1(Drive Request), Switch1/1
  PedalAccelValue/1 -> Totbereich Gaspedal/1(Pedal_Accel_Value)
  PedalBrakeRecuValue/1 -> Totbereich Bremspedal/1(Pedal_BrakeRecu_Value)
  Totbereich Bremspedal/1(BrakeTorque) -> Brake Map/1(BrakeTorque)
  Logical Operator1/1 -> Switch1/2
  Rate Transition/1 -> Brake Map/2(Driver)
  Rate Transition1/1 -> Subsystem/2(DrivingMode)

== system vd_controller/021_SignalProcessing/211_DriverSignalProcessing/DriverInput_Generation ==
  note: Der DrivingMode aus Inport 2 ist der, der beim Start ausgewählr wurde. Dieser wurde beim E9 in dem Block InverterInControl bestimmt und lässt sich während der Fahrt nicht ändern. Früher in die Funktionsstruktur integreireren, da so weniger umständlich.
  DriverInput_in : Inport
  DrivingMode : Inport  Port=2
  Bus Creator : BusCreator  Inputs=9
  Bus Selector : BusSelector  OutputSignals=db_PTM,db_button_low,vd_button_1,vd_button_2,vd_turnbutton_1,vd_turnbutton_2,driver,DriverInput_Sq
  DriverInput : Outport  VectorParamsAs1DForOutWhenUnconnected=off
  wires:
  DriverInput_in/1 -> Bus Selector/1
  Bus Creator/1 -> DriverInput/1  "DriverInput"
  Bus Selector/1 -> Bus Creator/1  "<db_PTM>"
  Bus Selector/2 -> Bus Creator/2  "<db_button_low>"
  Bus Selector/3 -> Bus Creator/3  "<vd_button_1>"
  Bus Selector/4 -> Bus Creator/4  "<vd_button_2>"
  Bus Selector/5 -> Bus Creator/5  "<vd_turnbutton_1>"
  Bus Selector/6 -> Bus Creator/6  "<vd_turnbutton_2>"
  Bus Selector/7 -> Bus Creator/7  "<driver>"
  DrivingMode/1 -> Bus Creator/9
  Bus Selector/8 -> Bus Creator/8  "<DriverInput_Sq>"

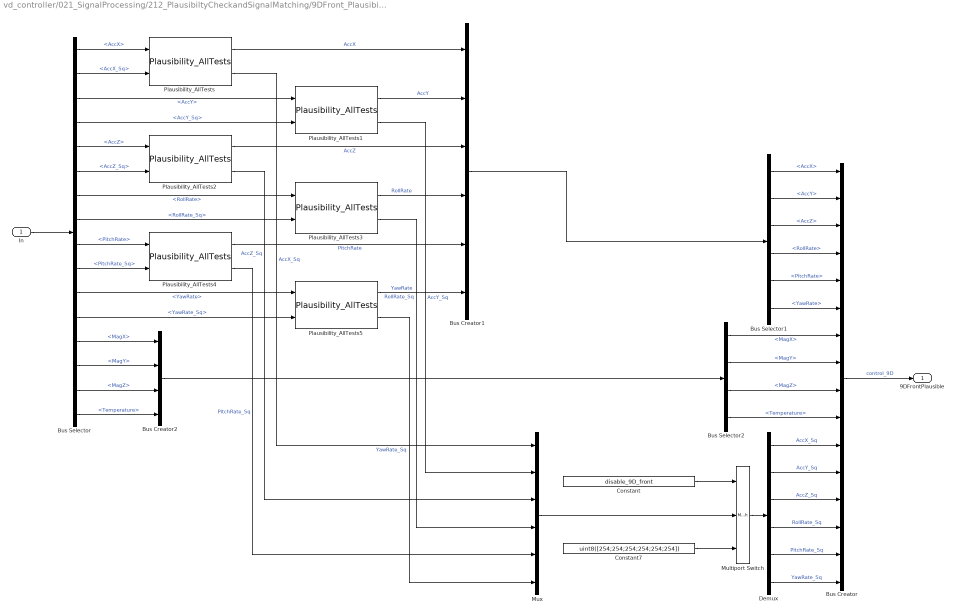
== system vd_controller/021_SignalProcessing/212_PlausibiltyCheckandSignalMatching/9DFront_Plausibility ==
  In : Inport  OutDataTypeStr=Bus: control_9D
  Bus Creator : BusCreator  Inputs=16  OutDataTypeStr=Bus: control_9D
  Bus Creator1 : BusCreator  Inputs=6
  Bus Creator2 : BusCreator  Inputs=4
  Bus Selector : BusSelector  OutputSignals=AccX,AccX_Sq,AccY,AccY_Sq,AccZ,AccZ_Sq,RollRate,RollRate_Sq,PitchRate,PitchRate_Sq,YawRate,YawRate_Sq,MagX,MagY,MagZ,Temperature
  Bus Selector1 : BusSelector  OutputSignals=AccX,AccY,AccZ,RollRate,PitchRate,YawRate
  Bus Selector2 : BusSelector  OutputSignals=MagX,MagY,MagZ,Temperature
  Constant : Constant  Value=disable_9D_front
  Constant7 : Constant  Value=uint8([254;254;254;254;254;254])
  Demux : Demux  Outputs=6
  Multiport Switch : MultiPortSwitch  DataPortOrder=Zero-based contiguous  Inputs=2  zeroidx=on
  Mux : Mux  Inputs=6
  Plausibility_AllTests : SignalProcessingSensorFusionLib/Plausibility_AllTests  alpha=0.3  checkGradient=off  deviation=0  threshold=0  alpha2=0  increasingPercentage=0  signalBounds=1e-8  stepDelay=25  upperBound=50  lowerBound=-50  useAlternativeValue=off  useManualAlternativeValue=off  manualAlternativeValue=0
  Plausibility_AllTests1 : SignalProcessingSensorFusionLib/Plausibility_AllTests  alpha=0.3  checkGradient=off  deviation=0  threshold=0  alpha2=0  increasingPercentage=0  signalBounds=1e-8  stepDelay=25  upperBound=50  lowerBound=-50  useAlternativeValue=off  useManualAlternativeValue=off  manualAlternativeValue=0
  Plausibility_AllTests2 : SignalProcessingSensorFusionLib/Plausibility_AllTests  alpha=0.3  checkGradient=off  deviation=0  threshold=0  alpha2=0  increasingPercentage=0  signalBounds=1e-8  stepDelay=25  upperBound=50  lowerBound=-50  useAlternativeValue=off  useManualAlternativeValue=off  manualAlternativeValue=0
  Plausibility_AllTests3 : SignalProcessingSensorFusionLib/Plausibility_AllTests  alpha=0.3  checkGradient=off  deviation=0  threshold=0  alpha2=0  increasingPercentage=0  signalBounds=1e-8  stepDelay=25  upperBound=1.6  lowerBound=-1.6  useAlternativeValue=off  useManualAlternativeValue=off  manualAlternativeValue=0
  Plausibility_AllTests4 : SignalProcessingSensorFusionLib/Plausibility_AllTests  alpha=0.3  checkGradient=off  deviation=0  threshold=0  alpha2=0  increasingPercentage=0  signalBounds=1e-8  stepDelay=25  upperBound=1.6  lowerBound=-1.6  useAlternativeValue=off  useManualAlternativeValue=off  manualAlternativeValue=0
  Plausibility_AllTests5 : SignalProcessingSensorFusionLib/Plausibility_AllTests  alpha=0.3  checkGradient=off  deviation=0  threshold=0  alpha2=0  increasingPercentage=0  signalBounds=1e-8  stepDelay=25  upperBound=1.6  lowerBound=-1.6  useAlternativeValue=off  useManualAlternativeValue=off  manualAlternativeValue=0
  9DFrontPlausible : Outport  VectorParamsAs1DForOutWhenUnconnected=off
  wires:
  Plausibility_AllTests1/1 -> Bus Creator1/2  "AccY"
  Bus Selector/3 -> Plausibility_AllTests1/1  "<AccY>"
  In/1 -> Bus Selector/1
  Plausibility_AllTests/1 -> Bus Creator1/1  "AccX"
  Bus Selector/1 -> Plausibility_AllTests/1  "<AccX>"
  Plausibility_AllTests2/1 -> Bus Creator1/3  "AccZ"
  Bus Selector/5 -> Plausibility_AllTests2/1  "<AccZ>"
  Bus Selector/7 -> Plausibility_AllTests3/1  "<RollRate>"
  Plausibility_AllTests3/1 -> Bus Creator1/4  "RollRate"
  Bus Creator/1 -> 9DFrontPlausible/1  "control_9D"
  Plausibility_AllTests4/1 -> Bus Creator1/5  "PitchRate"
  Plausibility_AllTests5/1 -> Bus Creator1/6  "YawRate"
  Bus Selector/9 -> Plausibility_AllTests4/1  "<PitchRate>"
  Bus Selector/11 -> Plausibility_AllTests5/1  "<YawRate>"
  Plausibility_AllTests5/2 -> Mux/6  "YawRate_Sq"
  Plausibility_AllTests4/2 -> Mux/5  "PitchRate_Sq"
  Plausibility_AllTests3/2 -> Mux/4  "RollRate_Sq"
  Plausibility_AllTests2/2 -> Mux/3  "AccZ_Sq"
  Plausibility_AllTests/2 -> Mux/1  "AccX_Sq"
  Plausibility_AllTests1/2 -> Mux/2  "AccY_Sq"
  Bus Selector/2 -> Plausibility_AllTests/2  "<AccX_Sq>"
  Bus Selector/4 -> Plausibility_AllTests1/2  "<AccY_Sq>"
  Bus Selector/6 -> Plausibility_AllTests2/2  "<AccZ_Sq>"
  Bus Selector/8 -> Plausibility_AllTests3/2  "<RollRate_Sq>"
  Bus Selector/10 -> Plausibility_AllTests4/2  "<PitchRate_Sq>"
  Bus Selector/12 -> Plausibility_AllTests5/2  "<YawRate_Sq>"
  Mux/1 -> Multiport Switch/2
  Constant7/1 -> Multiport Switch/3
  Multiport Switch/1 -> Demux/1
  Constant/1 -> Multiport Switch/1
  Demux/1 -> Bus Creator/11  "AccX_Sq"
  Demux/2 -> Bus Creator/12  "AccY_Sq"
  Demux/3 -> Bus Creator/13  "AccZ_Sq"
  Demux/4 -> Bus Creator/14  "RollRate_Sq"
  Demux/5 -> Bus Creator/15  "PitchRate_Sq"
  Demux/6 -> Bus Creator/16  "YawRate_Sq"
  Bus Creator1/1 -> Bus Selector1/1
  Bus Selector1/1 -> Bus Creator/1  "<AccX>"
  Bus Selector1/2 -> Bus Creator/2  "<AccY>"
  Bus Selector1/3 -> Bus Creator/3  "<AccZ>"
  Bus Selector1/4 -> Bus Creator/4  "<RollRate>"
  Bus Selector1/5 -> Bus Creator/5  "<PitchRate>"
  Bus Selector1/6 -> Bus Creator/6  "<YawRate>"
  Bus Selector/16 -> Bus Creator2/4  "<Temperature>"
  Bus Selector/15 -> Bus Creator2/3  "<MagZ>"
  Bus Selector/14 -> Bus Creator2/2  "<MagY>"
  Bus Selector/13 -> Bus Creator2/1  "<MagX>"
  Bus Creator2/1 -> Bus Selector2/1
  Bus Selector2/1 -> Bus Creator/7  "<MagX>"
  Bus Selector2/2 -> Bus Creator/8  "<MagY>"
  Bus Selector2/3 -> Bus Creator/9  "<MagZ>"
  Bus Selector2/4 -> Bus Creator/10  "<Temperature>"

== system vd_controller/021_SignalProcessing/212_PlausibiltyCheckandSignalMatching/9DRear_Plausibility ==
  In : Inport  OutDataTypeStr=Bus: control_9D
  Bus Creator1 : BusCreator  Inputs=16  OutDataTypeStr=Bus: control_9D
  Bus Creator2 : BusCreator  Inputs=6
  Bus Creator3 : BusCreator  Inputs=4
  Bus Selector1 : BusSelector  OutputSignals=AccX,AccX_Sq,AccY,AccY_Sq,AccZ,AccZ_Sq,RollRate,RollRate_Sq,PitchRate,PitchRate_Sq,YawRate,YawRate_Sq,MagX,MagY,MagZ,Temperature
  Bus Selector2 : BusSelector  OutputSignals=AccX,AccY,AccZ,RollRate,PitchRate,YawRate
  Bus Selector3 : BusSelector  OutputSignals=MagX,MagY,MagZ,Temperature
  Plausibility_AllTests10 : SignalProcessingSensorFusionLib/Plausibility_AllTests  alpha=0.3  checkGradient=off  deviation=0  threshold=0  alpha2=0  increasingPercentage=0  signalBounds=1e-8  stepDelay=25  upperBound=1.6  lowerBound=-1.6  useAlternativeValue=off  useManualAlternativeValue=off  manualAlternativeValue=0
  Plausibility_AllTests11 : SignalProcessingSensorFusionLib/Plausibility_AllTests  alpha=0.3  checkGradient=off  deviation=0  threshold=0  alpha2=0  increasingPercentage=0  signalBounds=1e-8  stepDelay=25  upperBound=1.6  lowerBound=-1.6  useAlternativeValue=off  useManualAlternativeValue=off  manualAlternativeValue=0
  Plausibility_AllTests6 : SignalProcessingSensorFusionLib/Plausibility_AllTests  alpha=0.3  checkGradient=off  deviation=0  threshold=0  alpha2=0  increasingPercentage=0  signalBounds=1e-8  stepDelay=25  upperBound=50  lowerBound=-50  useAlternativeValue=off  useManualAlternativeValue=off  manualAlternativeValue=0
  Plausibility_AllTests7 : SignalProcessingSensorFusionLib/Plausibility_AllTests  alpha=0.3  checkGradient=off  deviation=0  threshold=0  alpha2=0  increasingPercentage=0  signalBounds=1e-8  stepDelay=25  upperBound=50  lowerBound=-50  useAlternativeValue=off  useManualAlternativeValue=off  manualAlternativeValue=0
  Plausibility_AllTests8 : SignalProcessingSensorFusionLib/Plausibility_AllTests  alpha=0.3  checkGradient=off  deviation=0  threshold=0  alpha2=0  increasingPercentage=0  signalBounds=1e-8  stepDelay=25  upperBound=50  lowerBound=-50  useAlternativeValue=off  useManualAlternativeValue=off  manualAlternativeValue=0
  Plausibility_AllTests9 : SignalProcessingSensorFusionLib/Plausibility_AllTests  alpha=0.3  checkGradient=off  deviation=0  threshold=0  alpha2=0  increasingPercentage=0  signalBounds=1e-8  stepDelay=25  upperBound=1.6  lowerBound=-1.6  useAlternativeValue=off  useManualAlternativeValue=off  manualAlternativeValue=0
  9DRearPlausible : Outport  VectorParamsAs1DForOutWhenUnconnected=off
  wires:
  Bus Selector2/5 -> Bus Creator1/5  "<PitchRate>"
  Bus Selector1/15 -> Bus Creator3/3  "<MagZ>"
  Bus Selector1/14 -> Bus Creator3/2  "<MagY>"
  Bus Selector3/4 -> Bus Creator1/10  "<Temperature>"
  Bus Selector1/2 -> Plausibility_AllTests6/2  "<AccX_Sq>"
  Plausibility_AllTests10/2 -> Bus Creator1/15  "PitchRate_Sq"
  Bus Selector1/11 -> Plausibility_AllTests11/1  "<YawRate>"
  Bus Selector1/12 -> Plausibility_AllTests11/2  "<YawRate_Sq>"
  Bus Selector1/4 -> Plausibility_AllTests7/2  "<AccY_Sq>"
  Plausibility_AllTests7/2 -> Bus Creator1/12  "AccY_Sq"
  Plausibility_AllTests6/2 -> Bus Creator1/11  "AccX_Sq"
  Bus Selector1/8 -> Plausibility_AllTests9/2  "<RollRate_Sq>"
  Plausibility_AllTests9/2 -> Bus Creator1/14  "RollRate_Sq"
  Plausibility_AllTests11/2 -> Bus Creator1/16  "YawRate_Sq"
  Bus Selector1/6 -> Plausibility_AllTests8/2  "<AccZ_Sq>"
  Bus Selector1/10 -> Plausibility_AllTests10/2  "<PitchRate_Sq>"
  Bus Creator1/1 -> 9DRearPlausible/1  "control_9D"
  Bus Selector1/5 -> Plausibility_AllTests8/1  "<AccZ>"
  Bus Selector1/13 -> Bus Creator3/1  "<MagX>"
  Plausibility_AllTests8/2 -> Bus Creator1/13  "AccZ_Sq"
  In/1 -> Bus Selector1/1
  Bus Selector1/1 -> Plausibility_AllTests6/1  "<AccX>"
  Bus Selector1/3 -> Plausibility_AllTests7/1  "<AccY>"
  Bus Selector1/7 -> Plausibility_AllTests9/1  "<RollRate>"
  Bus Selector2/4 -> Bus Creator1/4  "<RollRate>"
  Bus Creator3/1 -> Bus Selector3/1
  Bus Selector2/2 -> Bus Creator1/2  "<AccY>"
  Bus Selector2/1 -> Bus Creator1/1  "<AccX>"
  Plausibility_AllTests7/1 -> Bus Creator2/2  "AccY"
  Bus Selector3/1 -> Bus Creator1/7  "<MagX>"
  Bus Selector3/3 -> Bus Creator1/9  "<MagZ>"
  Plausibility_AllTests8/1 -> Bus Creator2/3  "AccZ"
  Bus Selector2/6 -> Bus Creator1/6  "<YawRate>"
  Plausibility_AllTests6/1 -> Bus Creator2/1  "AccX"
  Bus Selector3/2 -> Bus Creator1/8  "<MagY>"
  Plausibility_AllTests11/1 -> Bus Creator2/6  "YawRate"
  Plausibility_AllTests10/1 -> Bus Creator2/5  "PitchRate"
  Bus Selector1/9 -> Plausibility_AllTests10/1  "<PitchRate>"
  Plausibility_AllTests9/1 -> Bus Creator2/4  "RollRate"
  Bus Selector2/3 -> Bus Creator1/3  "<AccZ>"
  Bus Selector1/16 -> Bus Creator3/4  "<Temperature>"
  Bus Creator2/1 -> Bus Selector2/1

== system vd_controller/021_SignalProcessing/212_PlausibiltyCheckandSignalMatching/DriverRequest_Plausibility ==
  In : Inport  OutDataTypeStr=Bus: control_DriverRequest
  Bus Creator : BusCreator  Inputs=11  OutDataTypeStr=Bus: control_DriverRequest
      settings: InheritFromInputs=off
  Bus Selector : BusSelector  OutputSignals=Pedal_BrakeMech_Value,Pedal_BrakeRecu_Value,SteeringwheelAngle,Pedal_Accel_Value,Pedal_TorqueValid_flag,Pedal_BrakeHard_flag,Pedal_BrakeMech_flag,SteeringValid_flag,Pedal_BrakeValid_flag,SteeringwheelAngle_Sq,Pedal_Accel_Value_Sq
  Data Type Conversion{1..3,6} (4 alike) : DataTypeConversion  OutDataTypeStr=uint8
  Data Type Conversion{4..5,7,9} (4 alike) : DataTypeConversion  OutDataTypeStr=single
  Plausibility_AllTests : SignalProcessingSensorFusionLib/Plausibility_AllTests  alpha=0.3  checkGradient=off  deviation=0  threshold=0  alpha2=0  increasingPercentage=0  signalBounds=1e-10  stepDelay=40  upperBound=120  lowerBound=-120  useAlternativeValue=off  useManualAlternativeValue=off  manualAlternativeValue=0
  Plausibility_AllTests1 : SignalProcessingSensorFusionLib/Plausibility_AllTests  alpha=0.3  checkGradient=off  deviation=0  threshold=0  alpha2=0  increasingPercentage=0  signalBounds=1e-10  stepDelay=40  upperBound=1  lowerBound=0  useAlternativeValue=off  useManualAlternativeValue=off  manualAlternativeValue=0
  DriverRequest : Outport  OutDataTypeStr=Bus: control_DriverRequest  VectorParamsAs1DForOutWhenUnconnected=off
  wires:
  In/1 -> Bus Selector/1
  Bus Creator/1 -> DriverRequest/1
  Bus Selector/1 -> Data Type Conversion7/1  "<Pedal_BrakeMech_Value>"
  Bus Selector/2 -> Data Type Conversion5/1  "<Pedal_BrakeRecu_Value>"
  Bus Selector/3 -> Plausibility_AllTests/1  "<SteeringwheelAngle>"
  Plausibility_AllTests/1 -> Data Type Conversion4/1  "SteeringwheelAngle"
  Bus Selector/4 -> Plausibility_AllTests1/1  "<Pedal_Accel_Value>"
  Bus Selector/5 -> Bus Creator/5  "<Pedal_TorqueValid_flag>"
  Bus Selector/6 -> Bus Creator/6  "<Pedal_BrakeHard_flag>"
  Bus Selector/7 -> Bus Creator/7  "<Pedal_BrakeMech_flag>"
  Bus Selector/8 -> Bus Creator/8  "<SteeringValid_flag>"
  Bus Selector/9 -> Bus Creator/9  "<Pedal_BrakeValid_flag>"
  Plausibility_AllTests/2 -> Data Type Conversion3/1  "SteeringwheelAngle_Sq"
  Plausibility_AllTests1/1 -> Data Type Conversion9/1  "Pedal_Accel_Value"
  Bus Selector/10 -> Data Type Conversion6/1  "<SteeringwheelAngle_Sq>"
  Data Type Conversion7/1 -> Bus Creator/1
  Data Type Conversion5/1 -> Bus Creator/2
  Data Type Conversion4/1 -> Bus Creator/3
  Data Type Conversion9/1 -> Bus Creator/4
  Bus Selector/11 -> Data Type Conversion1/1  "<Pedal_Accel_Value_Sq>"
  Plausibility_AllTests1/2 -> Data Type Conversion2/1  "Pedal_Accel_Value_Sq"
  Data Type Conversion2/1 -> Bus Creator/11
  Data Type Conversion6/1 -> Plausibility_AllTests/2
  Data Type Conversion1/1 -> Plausibility_AllTests1/2
  Data Type Conversion3/1 -> Bus Creator/10

== system vd_controller/021_SignalProcessing/212_PlausibiltyCheckandSignalMatching/Electric_Plausibility ==
  In : Inport  OutDataTypeStr=Bus: control_Electric
  Bus Creator : BusCreator  Inputs=12  OutDataTypeStr=Bus: control_Electric
  Bus Selector : BusSelector  OutputSignals=BatSOC,BatVoltage,BatPower,BatCurrent,AvgCellVoltage,MaxCellVoltage,MinCellVoltage,IVTEnergy,MinCellTemp,IVT_VoltageCurrent_Sq,IVT_Energy_Sq,HVM_BMS_Sq
  Data Type Conversion22 : DataTypeConversion  OutDataTypeStr=single
  Plausibility_AllTests : SignalProcessingSensorFusionLib/Plausibility_AllTests  alpha=0.5  checkGradient=off  deviation=0  threshold=0  alpha2=0  increasingPercentage=0  signalBounds=1e-10  stepDelay=40  upperBound=120000  lowerBound=-120000  useAlternativeValue=off  useManualAlternativeValue=off  manualAlternativeValue=0
  ElectricPlausible : Outport  VectorParamsAs1DForOutWhenUnconnected=off
  wires:
  Bus Selector/8 -> Plausibility_AllTests/1  "<IVTEnergy>"
  Bus Selector/7 -> Bus Creator/7  "<MinCellVoltage>"
  In/1 -> Bus Selector/1
  Bus Creator/1 -> ElectricPlausible/1  "Electric"
  Bus Selector/1 -> Bus Creator/1  "<BatSOC>"
  Bus Selector/2 -> Bus Creator/2  "<BatVoltage>"
  Bus Selector/3 -> Bus Creator/3  "<BatPower>"
  Bus Selector/4 -> Bus Creator/4  "<BatCurrent>"
  Bus Selector/5 -> Bus Creator/5  "<AvgCellVoltage>"
  Bus Selector/6 -> Bus Creator/6  "<MaxCellVoltage>"
  Bus Selector/9 -> Bus Creator/9  "<MinCellTemp>"
  Bus Selector/10 -> Bus Creator/10  "<IVT_VoltageCurrent_Sq>"
  Bus Selector/11 -> Plausibility_AllTests/2  "<IVT_Energy_Sq>"
  Bus Selector/12 -> Bus Creator/12  "<HVM_BMS_Sq>"
  Plausibility_AllTests/2 -> Bus Creator/11  "IVT_Energy_Sq"
  Plausibility_AllTests/1 -> Data Type Conversion22/1
  Data Type Conversion22/1 -> Bus Creator/8  "IVTEnergy"

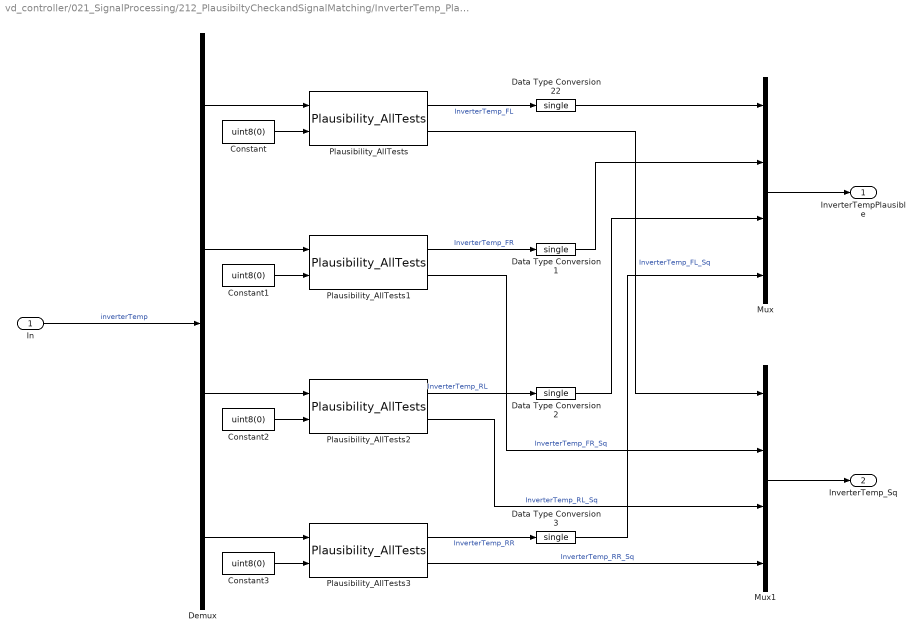
== system vd_controller/021_SignalProcessing/212_PlausibiltyCheckandSignalMatching/InverterTemp_Plausibility ==
  In : Inport  OutDataTypeStr=single  PortDimensions=4
  Constant{,1..3} (4 alike) : Constant  Value=uint8(0)
  Data Type Conversion{1..3,22} (4 alike) : DataTypeConversion  OutDataTypeStr=single
  Demux : Demux
  Mux : Mux
  Mux1 : Mux
  Plausibility_AllTests{,1..3} (4 alike) : SignalProcessingSensorFusionLib/Plausibility_AllTests  alpha=0.5  checkGradient=off  deviation=0  threshold=0  alpha2=0  increasingPercentage=0  signalBounds=1e-12  stepDelay=40  upperBound=75  lowerBound=-10  useAlternativeValue=off  useManualAlternativeValue=off  manualAlternativeValue=0
  InverterTempPlausible : Outport  VectorParamsAs1DForOutWhenUnconnected=off
  InverterTemp_Sq : Outport  Port=2  VectorParamsAs1DForOutWhenUnconnected=off
  wires:
  Plausibility_AllTests1/1 -> Data Type Conversion1/1  "InverterTemp_FR"
  In/1 -> Demux/1  "inverterTemp"
  Plausibility_AllTests/1 -> Data Type Conversion22/1  "InverterTemp_FL"
  Plausibility_AllTests2/1 -> Data Type Conversion2/1  "InverterTemp_RL"
  Demux/1 -> Plausibility_AllTests/1
  Demux/2 -> Plausibility_AllTests1/1
  Demux/3 -> Plausibility_AllTests2/1
  Plausibility_AllTests2/2 -> Mux1/3  "InverterTemp_RL_Sq"
  Plausibility_AllTests1/2 -> Mux1/2  "InverterTemp_FR_Sq"
  Demux/4 -> Plausibility_AllTests3/1
  Constant/1 -> Plausibility_AllTests/2
  Constant1/1 -> Plausibility_AllTests1/2
  Constant2/1 -> Plausibility_AllTests2/2
  Constant3/1 -> Plausibility_AllTests3/2
  Plausibility_AllTests3/1 -> Data Type Conversion3/1  "InverterTemp_RR"
  Mux/1 -> InverterTempPlausible/1
  Mux1/1 -> InverterTemp_Sq/1
  Plausibility_AllTests3/2 -> Mux1/4  "InverterTemp_RR_Sq"
  Plausibility_AllTests/2 -> Mux1/1  "InverterTemp_FL_Sq"
  Data Type Conversion22/1 -> Mux/1
  Data Type Conversion1/1 -> Mux/2
  Data Type Conversion2/1 -> Mux/3
  Data Type Conversion3/1 -> Mux/4
